simulink model "ersteSteuerung"  (R2016b)
settings: Solver=VariableStepAuto  StartTime=0.0  StopTime=inf  RelTol=1e-3
settings Model: Creator=hutte  LastModifiedBy=Patrick

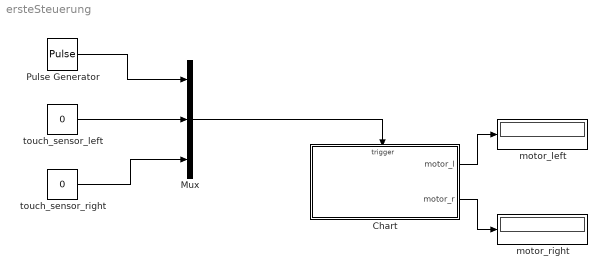
== system ersteSteuerung ==
  Chart : Stateflow chart  TreatAsAtomicUnit=on
  Mux : Mux  Inputs=3
  Pulse Generator : DiscretePulseGenerator  PulseType=Time based  Period=10  PulseWidth=5
  motor_left : Display
  motor_right : Display
  "touch_sensor_left " : Constant  Value=0
  "touch_sensor_right " : Constant  Value=0
  wires:
  "touch_sensor_left "/1 -> Mux/2
  "touch_sensor_right "/1 -> Mux/3
  Mux/1 -> Chart/Trigger
  Chart/1(motor_l) -> motor_left/1
  Chart/2(motor_r) -> motor_right/1
  Pulse Generator/1 -> Mux/1

== stateflow chart ersteSteuerung/Chart ==
  state FORWARD
    entry:
    motor_l=1;
    motor_r=1;
  state TURN_LEFT
    entry:
    motor_l=2;
    motor_r=1;
  state TURN_RIGHT
    entry:
    motor_l=1;
    motor_r=2;
  state BACKWARD
    entry:
    motor_l=2;
    motor_r=2;
    state LEFT
    state RIGHT
    (default) -> RIGHT
  (default) -> FORWARD
  TURN_RIGHT -> FORWARD : after(3, sec)
  TURN_LEFT -> FORWARD : after(3, sec)
  FORWARD -> LEFT [order 1] : touch_sensor_left
  FORWARD -> RIGHT [order 2] : touch_sensor_right
  LEFT -> TURN_LEFT : after(2, sec)
  RIGHT -> TURN_RIGHT : after(2, sec)
  data: motor_l output; motor_r output
  events: touch_sensor_left input RISING_EDGE_EVENT; touch_sensor_right input RISING_EDGE_EVENT; clk input RISING_EDGE_EVENT
